simulink model "full_maneuver_platoon"  (R2022a)
settings: Solver=ode23t  StartTime=0.0  StopTime=300  FixedStep=0.1  MaxStep=0.01  RelTol=1e-3
InitFcn:
  | totalVehicles = 7;
  | if exist('vehStatesBus', 'var')==0
  | load vehBuses
  | end
  | if exist('vehErrorsBus', 'var')==0
  | load vehBuses
  | end
libraries: simulink x80, powerlib_meascontrol x16, autolibshared x7, dspsigops x4
(part 1 of 9)
settings Model: Creator=fvall  LastModifiedBy=fvall
settings SolverCC: AlgebraicLoopSolver=TrustRegion
settings DebuggingCC: ReadBeforeWriteMsg=DisableAll  WriteAfterWriteMsg=DisableAll  WriteAfterReadMsg=DisableAll  MultiTaskDSMMsg=none  UnconnectedInputMsg=warning  UnconnectedOutputMsg=warning  UnconnectedLineMsg=warning  SFMachineParentedDataDiag=warning
settings ModelReferenceCC: UpdateModelReferenceTargets=IfOutOfDate
settings SFSimCC: SFSimEcho=off  CustomCodeUndefinedFunction=UseInterfaceOnly

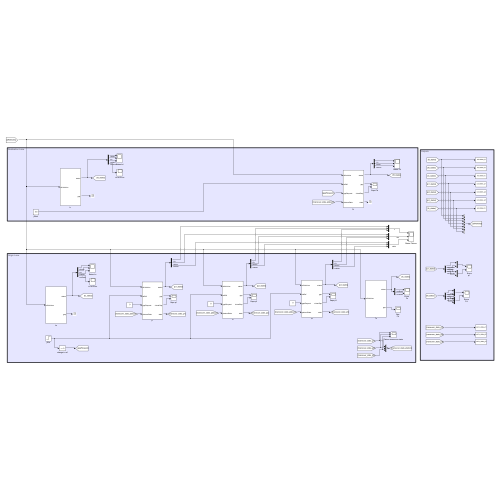
[thumbnail: Simulink's stored preview of the top-level diagram]
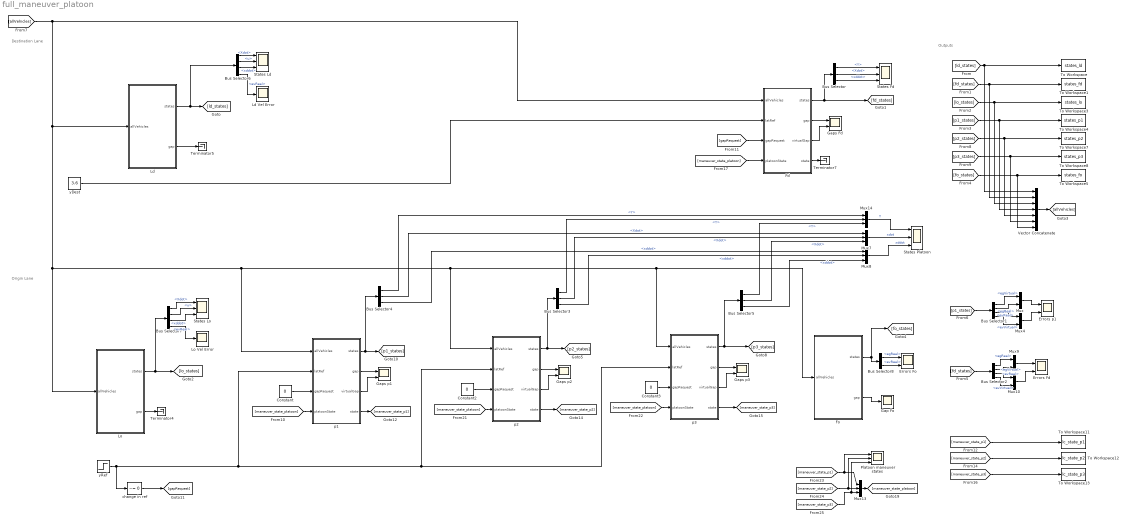
== system full_maneuver_platoon ==
  note: Destination Lane
  note: Outputs
  note: Origin Lane
  Bus Selector{,3..5} (4 alike) : BusSelector  OutputSignals=Y,Xdot,xddot
  Bus Selector1 : BusSelector  OutputSignals=egVirtual,egReal,evReal,evVirtual
  Bus Selector2 : BusSelector  OutputSignals=egReal,egVirtual,evReal,evVirtual
  Bus Selector6 : BusSelector  OutputSignals=Xdot,u,xddot,evReal
  Bus Selector7 : BusSelector  OutputSignals=Xdot,u,xddot,evReal
  Bus Selector8 : BusSelector  OutputSignals=egReal,evReal
  Constant : Constant  Value=0
  Constant2 : Constant  Value=0
  Constant3 : Constant  Value=0
  Errors Fd : Scope  NumInputPorts=2
  Errors Fo : Scope  NumInputPorts=2
  Errors p1 : Scope  NumInputPorts=2
  Fd : Subsystem  mask{m=2000, lf=2.5, lr=2.5, maxAcceleration=3, minAcceleration=-8, maxJerk=50, minJerk=-50, maxDelta=0.43633, maxDeltaDot=0.16406, freeFlowVel=30, posInPlatoon=1, tau=0.5, A=[0 1 20 0;0 -2.3 0 -21.4;0 0 0 1;0 -0.7 0 -7.6], B=[0;24;0;36], C=[1 0 0 0;0 1 0 0;0 0 1 0;0 0 0 1], x0=129.8137, vx0=25, y0=3.6, h=2.1778, d0=0.01134, minGapError=-100, maxGapError=Inf, velFilterGain=10, Kd=0.45918, Kp=0.045918, Ki=0, Ka=0.25255, Kdd=0.025255, velKi=0.11304, velKp=0.54492, velKd=0.07454, hFilterGain=0.3, hFilterSaturation=Inf, vMin=16.25, maxComfAccel=0.5, minComfAccel=-0.5, maxComfJerk=10, minComfJerk=-10, strategyChoice=leaderFirstInvert, hLC=2.2978, d0LC=0.01134, Klat=[0.0363636363636331 0.000980533179898461 1.32121212121203 0.0854574223245029], L=[3 1 20 0;0 3.7 0 -21.4;0 0 12 1;0 -0.7 0 10.4]}
      mask prompts: m "autoblks_shared:autoblkVehBody3DofLat:blkPrm_m"; lf "autoblks_shared:autoblkVehBody3DofLat:blkPrm_a"; lr "autoblks_shared:autoblkVehBody3DofLat:blkPrm_b"; maxAcceleration "Max Acceleration"; minAcceleration "Min Acceleration"; maxJerk "Max Jerk"; minJerk "Min Jerk"; maxDelta "Max Delta"; maxDeltaDot "Max Delta Dot"; freeFlowVel "Free Flow Velocity"; posInPlatoon "Position in Platoon"; tau "Actuator Lag"; x0 "autoblks_shared:autoblkVehBody3DofLat:blkPrm_X_o"; vx0 "autoblks_shared:autoblkVehBody3DofLat:blkPrm_xdot_o"; y0 "autoblks_shared:autoblkVehBody3DofLat:blkPrm_Y_o"; h "Time Headway"; d0 "Standstill Gap"; minGapError "Min Gap Error"; maxGapError "Max Gap Error"; velFilterGain "Velocity Filter Gain"; hFilterGain "Headway Filter Gain"; hFilterSaturation "Headway Filter Saturation"; vMin "Min Velocity"; maxComfAccel "Max Comf Accel"; minComfAccel "Min Comf Accel"; maxComfJerk "Max Comf Jerk"; minComfJerk "Min Comf Jerk"; strategyChoice "Lane Change Strategy"; hLC "Time Headway LC"; d0LC "Standstill Gap LC"; Klat "Lat Controller Gain"; L "Observer Gain"
      mask TypeOptions m: Vehicle Body 3DOF Single Track/m
      mask TypeOptions lf: Vehicle Body 3DOF Single Track/a
      mask TypeOptions lr: Vehicle Body 3DOF Single Track/b
      mask TypeOptions maxDelta: Lateral Control/Saturation/UpperLimit
      mask TypeOptions maxDeltaDot: Lateral Control/Rate Limiter/RisingSlewLimit
      mask TypeOptions posInPlatoon: posInPlatoon/Value
      mask TypeOptions A:
      | Lateral Control/Full State
      | Observer/Gain3/Gain
      mask TypeOptions B:
      | Lateral Control/Full State
      | Observer/Gain/Gain
      mask TypeOptions C:
      | Lateral Control/Full State
      | Observer/Gain1/Gain
      mask TypeOptions x0: Vehicle Body 3DOF Single Track/X_o
      mask TypeOptions vx0: Vehicle Body 3DOF Single Track/xdot_o
      mask TypeOptions y0: Vehicle Body 3DOF Single Track/Y_o
      mask TypeOptions strategyChoice: Lane Change Strategy/LabelModeActiveChoice
      mask TypeOptions Klat: Lateral Control/Gain1/Gain
      mask TypeOptions L:
      | Lateral Control/Full State
      | Observer/Gain2/Gain
      mask DialogControl DescGroupVar Prompt: 3DOF Vehicle with ACC
      mask DialogControl DescTextVar Prompt: Vehicle with ACC. The vehicle model is Simulink's 3DOF single track vehicle body. The controller is a PID with constant headway including headway error saturation and filtered leader velocity.
      mask DialogControl VehParams Prompt: Vehicle Parameters
      mask DialogControl m Prompt: Vehicle mass, m [kg]:
      mask DialogControl lf Prompt: Longitudinal distance from center of mass to front axle, a [m]:
      mask DialogControl lr Prompt: Longitudinal distance from center of mass to rear axle, b [m]:
      mask DialogControl latLinearModel Prompt: Lat Linear Model
      mask DialogControl InitStates Prompt: Initial State
      mask DialogControl x0 Prompt: Initial inertial frame longitudinal position, X_o [m]:
      mask DialogControl vx0 Prompt: Initial longitudinal velocity, xdot_o [m/s]:
      mask DialogControl y0 Prompt: Initial inertial frame lateral displacement, Y_o [m]:
      mask DialogControl Container3 Prompt: Veh Following Parameters
      mask DialogControl ComfortConstraints Prompt: Comfort Constraints
      mask DialogControl LCParams Prompt: Lane Change Params
  Fo : Subsystem  mask{m=2000, lf=2.5, lr=2.5, maxAcceleration=3, minAcceleration=-8, maxJerk=50, minJerk=-50, freeFlowVel=30, tau=0.5, x0=0, vx0=20, y0=0, h=2.1778, d0=0.01134, minGapError=-100, maxGapError=Inf, velFilterGain=10, Kd=0.45918, Kp=0.045918, Ki=0, Ka=0.25255, Kdd=0.025255, velKi=0.11304, velKp=0.54492, velKd=0.07454, hFilterGain=0.3, hFilterSaturation=Inf, vMin=13, maxComfAccel=0.5, minComfAccel=-0.5, maxComfJerk=10, minComfJerk=-10, hLC=2.2978, d0LC=0.01134}
      mask prompts: m "autoblks_shared:autoblkVehBody3DofLat:blkPrm_m"; lf "autoblks_shared:autoblkVehBody3DofLat:blkPrm_a"; lr "autoblks_shared:autoblkVehBody3DofLat:blkPrm_b"; maxAcceleration "Max Acceleration"; minAcceleration "Min Acceleration"; maxJerk "Max Jerk"; minJerk "Min Jerk"; freeFlowVel "Free Flow Velocity"; tau "Actuator Lag"; x0 "autoblks_shared:autoblkVehBody3DofLat:blkPrm_X_o"; vx0 "autoblks_shared:autoblkVehBody3DofLat:blkPrm_xdot_o"; y0 "autoblks_shared:autoblkVehBody3DofLat:blkPrm_Y_o"; h "Time Headway"; d0 "Standstill Gap"; minGapError "Min Gap Error"; maxGapError "Max Gap Error"; velFilterGain "Velocity Filter Gain"; hFilterGain "Headway Filter Gain"; hFilterSaturation "Headway Filter Saturation"; vMin "Min Velocity"; maxComfAccel "Max Comf Accel"; minComfAccel "Min Comf Accel"; maxComfJerk "Max Comf Jerk"; minComfJerk "Min Comf Jerk"; hLC "Time Headway LC"; d0LC "Standstill Gap LC"
      mask TypeOptions m: Vehicle Body 3DOF Single Track/m
      mask TypeOptions lf: Vehicle Body 3DOF Single Track/a
      mask TypeOptions lr: Vehicle Body 3DOF Single Track/b
      mask TypeOptions x0: Vehicle Body 3DOF Single Track/X_o
      mask TypeOptions vx0: Vehicle Body 3DOF Single Track/xdot_o
      mask TypeOptions y0: Vehicle Body 3DOF Single Track/Y_o
      mask DialogControl DescGroupVar Prompt: 3DOF Vehicle with ACC
      mask DialogControl DescTextVar Prompt: Vehicle with ACC. The vehicle model is Simulink's 3DOF single track vehicle body. The controller is a PID with constant headway including headway error saturation and filtered leader velocity.
      mask DialogControl VehParams Prompt: Vehicle Parameters
      mask DialogControl m Prompt: Vehicle mass, m [kg]:
      mask DialogControl lf Prompt: Longitudinal distance from center of mass to front axle, a [m]:
      mask DialogControl lr Prompt: Longitudinal distance from center of mass to rear axle, b [m]:
      mask DialogControl InitStates Prompt: Initial State
      mask DialogControl x0 Prompt: Initial inertial frame longitudinal position, X_o [m]:
      mask DialogControl vx0 Prompt: Initial longitudinal velocity, xdot_o [m/s]:
      mask DialogControl y0 Prompt: Initial inertial frame lateral displacement, Y_o [m]:
      mask DialogControl Container3 Prompt: Veh Following Parameters
      mask DialogControl ComfortConstraints Prompt: Comfort Constraints
      mask DialogControl LaneChangeParams Prompt: Lane Change Params
  Gap Fo : Scope
  Gaps Fd : Scope  NumInputPorts=2
  Gaps p1 : Scope  NumInputPorts=2
  Gaps p2 : Scope  NumInputPorts=2
  Gaps p3 : Scope  NumInputPorts=2
  Ld : Subsystem  mask{m=2000, lf=2.5, lr=2.5, maxAcceleration=3, minAcceleration=-8, maxJerk=50, minJerk=-50, freeFlowVel=25, tau=0.5, x0=189.2704, vx0=25, y0=3.6, h=0.30281, d0=0.01134, minGapError=-100, maxGapError=Inf, velFilterGain=10, Kd=3.3024, Kp=0.33024, Ki=0, Ka=1.8163, Kdd=0.18163, velKi=0.11304, velKp=0.54492, velKd=0.07454, hFilterGain=0.3, hFilterSaturation=Inf, vMin=16.25, maxComfAccel=0.5, minComfAccel=-0.5, maxComfJerk=10, minComfJerk=-10, hLC=1.8025, d0LC=0.01134}
      mask prompts: m "autoblks_shared:autoblkVehBody3DofLat:blkPrm_m"; lf "autoblks_shared:autoblkVehBody3DofLat:blkPrm_a"; lr "autoblks_shared:autoblkVehBody3DofLat:blkPrm_b"; maxAcceleration "Max Acceleration"; minAcceleration "Min Acceleration"; maxJerk "Max Jerk"; minJerk "Min Jerk"; freeFlowVel "Free Flow Velocity"; tau "Actuator Lag"; x0 "autoblks_shared:autoblkVehBody3DofLat:blkPrm_X_o"; vx0 "autoblks_shared:autoblkVehBody3DofLat:blkPrm_xdot_o"; y0 "autoblks_shared:autoblkVehBody3DofLat:blkPrm_Y_o"; h "Time Headway"; d0 "Standstill Gap"; minGapError "Min Gap Error"; maxGapError "Max Gap Error"; velFilterGain "Velocity Filter Gain"; hFilterGain "Headway Filter Gain"; hFilterSaturation "Headway Filter Saturation"; vMin "Min Velocity"; maxComfAccel "Max Comf Accel"; minComfAccel "Min Comf Accel"; maxComfJerk "Max Comf Jerk"; minComfJerk "Min Comf Jerk"; hLC "Time Headway LC"; d0LC "Standstill Gap LC"
      mask TypeOptions m: Vehicle Body 3DOF Single Track/m
      mask TypeOptions lf: Vehicle Body 3DOF Single Track/a
      mask TypeOptions lr: Vehicle Body 3DOF Single Track/b
      mask TypeOptions x0: Vehicle Body 3DOF Single Track/X_o
      mask TypeOptions vx0: Vehicle Body 3DOF Single Track/xdot_o
      mask TypeOptions y0: Vehicle Body 3DOF Single Track/Y_o
      mask DialogControl DescGroupVar Prompt: 3DOF Vehicle with ACC
      mask DialogControl DescTextVar Prompt: Vehicle with ACC. The vehicle model is Simulink's 3DOF single track vehicle body. The controller is a PID with constant headway including headway error saturation and filtered leader velocity.
      mask DialogControl VehParams Prompt: Vehicle Parameters
      mask DialogControl m Prompt: Vehicle mass, m [kg]:
      mask DialogControl lf Prompt: Longitudinal distance from center of mass to front axle, a [m]:
      mask DialogControl lr Prompt: Longitudinal distance from center of mass to rear axle, b [m]:
      mask DialogControl InitStates Prompt: Initial State
      mask DialogControl x0 Prompt: Initial inertial frame longitudinal position, X_o [m]:
      mask DialogControl vx0 Prompt: Initial longitudinal velocity, xdot_o [m/s]:
      mask DialogControl y0 Prompt: Initial inertial frame lateral displacement, Y_o [m]:
      mask DialogControl Container3 Prompt: Veh Following Parameters
      mask DialogControl ComfortConstraints Prompt: Comfort Constraints
      mask DialogControl LaneChangeParams Prompt: Lane Change Params
  Ld Vel Error : Scope
  Lo : Subsystem  mask{m=2000, lf=2.5, lr=2.5, maxAcceleration=3, minAcceleration=-8, maxJerk=50, minJerk=-50, freeFlowVel=20, tau=0.5, x0=194.2704, vx0=20, y0=0, h=0.30281, d0=0.01134, minGapError=-100, maxGapError=Inf, velFilterGain=10, Kd=3.3024, Kp=0.33024, Ki=0, Ka=1.8163, Kdd=0.18163, velKi=0.11304, velKp=0.54492, velKd=0.07454, hFilterGain=0.3, hFilterSaturation=Inf, vMin=13, maxComfAccel=0.5, minComfAccel=-0.5, maxComfJerk=10, minComfJerk=-10, hLC=1.49, d0LC=0.01134}
      mask prompts: m "autoblks_shared:autoblkVehBody3DofLat:blkPrm_m"; lf "autoblks_shared:autoblkVehBody3DofLat:blkPrm_a"; lr "autoblks_shared:autoblkVehBody3DofLat:blkPrm_b"; maxAcceleration "Max Acceleration"; minAcceleration "Min Acceleration"; maxJerk "Max Jerk"; minJerk "Min Jerk"; freeFlowVel "Free Flow Velocity"; tau "Actuator Lag"; x0 "autoblks_shared:autoblkVehBody3DofLat:blkPrm_X_o"; vx0 "autoblks_shared:autoblkVehBody3DofLat:blkPrm_xdot_o"; y0 "autoblks_shared:autoblkVehBody3DofLat:blkPrm_Y_o"; h "Time Headway"; d0 "Standstill Gap"; minGapError "Min Gap Error"; maxGapError "Max Gap Error"; velFilterGain "Velocity Filter Gain"; hFilterGain "Headway Filter Gain"; hFilterSaturation "Headway Filter Saturation"; vMin "Min Velocity"; maxComfAccel "Max Comf Accel"; minComfAccel "Min Comf Accel"; maxComfJerk "Max Comf Jerk"; minComfJerk "Min Comf Jerk"; hLC "Time Headway LC"; d0LC "Standstill Gap LC"
      mask TypeOptions m: Vehicle Body 3DOF Single Track/m
      mask TypeOptions lf: Vehicle Body 3DOF Single Track/a
      mask TypeOptions lr: Vehicle Body 3DOF Single Track/b
      mask TypeOptions x0: Vehicle Body 3DOF Single Track/X_o
      mask TypeOptions vx0: Vehicle Body 3DOF Single Track/xdot_o
      mask TypeOptions y0: Vehicle Body 3DOF Single Track/Y_o
      mask DialogControl DescGroupVar Prompt: 3DOF Vehicle with ACC
      mask DialogControl DescTextVar Prompt: Vehicle with ACC. The vehicle model is Simulink's 3DOF single track vehicle body. The controller is a PID with constant headway including headway error saturation and filtered leader velocity.
      mask DialogControl VehParams Prompt: Vehicle Parameters
      mask DialogControl m Prompt: Vehicle mass, m [kg]:
      mask DialogControl lf Prompt: Longitudinal distance from center of mass to front axle, a [m]:
      mask DialogControl lr Prompt: Longitudinal distance from center of mass to rear axle, b [m]:
      mask DialogControl InitStates Prompt: Initial State
      mask DialogControl x0 Prompt: Initial inertial frame longitudinal position, X_o [m]:
      mask DialogControl vx0 Prompt: Initial longitudinal velocity, xdot_o [m/s]:
      mask DialogControl y0 Prompt: Initial inertial frame lateral displacement, Y_o [m]:
      mask DialogControl Container3 Prompt: Veh Following Parameters
      mask DialogControl ComfortConstraints Prompt: Comfort Constraints
      mask DialogControl LaneChangeParams Prompt: Lane Change Params
  Lo Vel Error : Scope
  Mux{,4,9..10} (4 alike) : Mux  Inputs=2
  Mux{7..8,13..14} (4 alike) : Mux  Inputs=3
  Platoon maneuver states : Scope  NumInputPorts=3
  States Fd : Scope  NumInputPorts=3
  States Ld : Scope  NumInputPorts=3
  States Lo : Scope  NumInputPorts=3
  States Platoon : Scope  NumInputPorts=3
  Terminator4 : Terminator
  Terminator5 : Terminator
  Terminator7 : Terminator
  To Workspace : ToWorkspace  VariableName=states_ld  SaveFormat=Timeseries  SampleTime=-1
  To Workspace1 : ToWorkspace  VariableName=states_fd  SaveFormat=Timeseries  SampleTime=-1
  To Workspace11 : ToWorkspace  VariableName=lc_state_p1  SaveFormat=Timeseries  SampleTime=-1
  To Workspace12 : ToWorkspace  VariableName=lc_state_p2  SaveFormat=Timeseries  SampleTime=-1
  To Workspace13 : ToWorkspace  VariableName=lc_state_p3  SaveFormat=Timeseries  SampleTime=-1
  To Workspace3 : ToWorkspace  VariableName=states_lo  SaveFormat=Timeseries  SampleTime=-1
  To Workspace4 : ToWorkspace  VariableName=states_p1  SaveFormat=Timeseries  SampleTime=-1
  To Workspace5 : ToWorkspace  VariableName=states_fo  SaveFormat=Timeseries  SampleTime=-1
  To Workspace7 : ToWorkspace  VariableName=states_p2  SaveFormat=Timeseries  SampleTime=-1
  To Workspace8 : ToWorkspace  VariableName=states_p3  SaveFormat=Timeseries  SampleTime=-1
  Vector Concatenate : Concatenate  NumInputs=7
  change in ref : simulink/Logic and Bit Operations/Compare To Constant  relop=~=  const=0  OutDataTypeStr=boolean
  p1 : Subsystem  mask{m=2000, lf=2.5, lr=2.5, maxAcceleration=3, minAcceleration=-8, maxJerk=50, minJerk=-50, maxDelta=0.43633, maxDeltaDot=0.16406, freeFlowVel=30, posInPlatoon=1, tau=0.5, A=[0 1 20 0;0 -2.3 0 -21.4;0 0 0 1;0 -0.7 0 -7.6], B=[0;24;0;36], C=[1 0 0 0;0 1 0 0;0 0 1 0;0 0 0 1], x0=145.7028, vx0=20, y0=0, h=2.1778, d0=0.01134, minGapError=-100, maxGapError=Inf, velFilterGain=10, Kd=0.45918, Kp=0.045918, Ki=0, Ka=0.25255, Kdd=0.025255, velKi=0.11304, velKp=0.54492, velKd=0.07454, hFilterGain=0.3, hFilterSaturation=Inf, vMin=13, maxComfAccel=0.5, minComfAccel=-0.5, maxComfJerk=10, minComfJerk=-10, strategyChoice=leaderFirstInvert, hLC=2.2978, d0LC=0.01134, Klat=[0.0363636363636331 0.000980533179898461 1.32121212121203 0.0854574223245029], L=[3 1 20 0;0 3.7 0 -21.4;0 0 12 1;0 -0.7 0 10.4]}
      mask prompts: m "autoblks_shared:autoblkVehBody3DofLat:blkPrm_m"; lf "autoblks_shared:autoblkVehBody3DofLat:blkPrm_a"; lr "autoblks_shared:autoblkVehBody3DofLat:blkPrm_b"; maxAcceleration "Max Acceleration"; minAcceleration "Min Acceleration"; maxJerk "Max Jerk"; minJerk "Min Jerk"; maxDelta "Max Delta"; maxDeltaDot "Max Delta Dot"; freeFlowVel "Free Flow Velocity"; posInPlatoon "Position in Platoon"; tau "Actuator Lag"; x0 "autoblks_shared:autoblkVehBody3DofLat:blkPrm_X_o"; vx0 "autoblks_shared:autoblkVehBody3DofLat:blkPrm_xdot_o"; y0 "autoblks_shared:autoblkVehBody3DofLat:blkPrm_Y_o"; h "Time Headway"; d0 "Standstill Gap"; minGapError "Min Gap Error"; maxGapError "Max Gap Error"; velFilterGain "Velocity Filter Gain"; hFilterGain "Headway Filter Gain"; hFilterSaturation "Headway Filter Saturation"; vMin "Min Velocity"; maxComfAccel "Max Comf Accel"; minComfAccel "Min Comf Accel"; maxComfJerk "Max Comf Jerk"; minComfJerk "Min Comf Jerk"; strategyChoice "Lane Change Strategy"; hLC "Time Headway LC"; d0LC "Standstill Gap LC"; Klat "Lat Controller Gain"; L "Observer Gain"
      mask TypeOptions m: Vehicle Body 3DOF Single Track/m
      mask TypeOptions lf: Vehicle Body 3DOF Single Track/a
      mask TypeOptions lr: Vehicle Body 3DOF Single Track/b
      mask TypeOptions maxDelta: Lateral Control/Saturation/UpperLimit
      mask TypeOptions maxDeltaDot: Lateral Control/Rate Limiter/RisingSlewLimit
      mask TypeOptions posInPlatoon: posInPlatoon/Value
      mask TypeOptions A:
      | Lateral Control/Full State
      | Observer/Gain3/Gain
      mask TypeOptions B:
      | Lateral Control/Full State
      | Observer/Gain/Gain
      mask TypeOptions C:
      | Lateral Control/Full State
      | Observer/Gain1/Gain
      mask TypeOptions x0: Vehicle Body 3DOF Single Track/X_o
      mask TypeOptions vx0: Vehicle Body 3DOF Single Track/xdot_o
      mask TypeOptions y0: Vehicle Body 3DOF Single Track/Y_o
      mask TypeOptions strategyChoice: Lane Change Strategy/LabelModeActiveChoice
      mask TypeOptions Klat: Lateral Control/Gain1/Gain
      mask TypeOptions L:
      | Lateral Control/Full State
      | Observer/Gain2/Gain
      mask DialogControl DescGroupVar Prompt: 3DOF Vehicle with ACC
      mask DialogControl DescTextVar Prompt: Vehicle with ACC. The vehicle model is Simulink's 3DOF single track vehicle body. The controller is a PID with constant headway including headway error saturation and filtered leader velocity.
      mask DialogControl VehParams Prompt: Vehicle Parameters
      mask DialogControl m Prompt: Vehicle mass, m [kg]:
      mask DialogControl lf Prompt: Longitudinal distance from center of mass to front axle, a [m]:
      mask DialogControl lr Prompt: Longitudinal distance from center of mass to rear axle, b [m]:
      mask DialogControl latLinearModel Prompt: Lat Linear Model
      mask DialogControl InitStates Prompt: Initial State
      mask DialogControl x0 Prompt: Initial inertial frame longitudinal position, X_o [m]:
      mask DialogControl vx0 Prompt: Initial longitudinal velocity, xdot_o [m/s]:
      mask DialogControl y0 Prompt: Initial inertial frame lateral displacement, Y_o [m]:
      mask DialogControl Container3 Prompt: Veh Following Parameters
      mask DialogControl ComfortConstraints Prompt: Comfort Constraints
      mask DialogControl LCParams Prompt: Lane Change Params
  p2 : Subsystem  mask{m=2000, lf=2.5, lr=2.5, maxAcceleration=3, minAcceleration=-8, maxJerk=50, minJerk=-50, maxDelta=0.43633, maxDeltaDot=0.16406, freeFlowVel=30, posInPlatoon=2, tau=0.5, A=[0 1 20 0;0 -2.3 0 -21.4;0 0 0 1;0 -0.7 0 -7.6], B=[0;24;0;36], C=[1 0 0 0;0 1 0 0;0 0 1 0;0 0 0 1], x0=97.1352, vx0=20, y0=0, h=2.1778, d0=0.01134, minGapError=-100, maxGapError=Inf, velFilterGain=10, Kd=0.45918, Kp=0.045918, Ki=0, Ka=0.25255, Kdd=0.025255, velKi=0.11304, velKp=0.54492, velKd=0.07454, hFilterGain=0.3, hFilterSaturation=Inf, vMin=13, maxComfAccel=0.5, minComfAccel=-0.5, maxComfJerk=10, minComfJerk=-10, strategyChoice=leaderFirstInvert, hLC=2.2978, d0LC=0.01134, Klat=[0.0363636363636331 0.000980533179898461 1.32121212121203 0.0854574223245029], L=[3 1 20 0;0 3.7 0 -21.4;0 0 12 1;0 -0.7 0 10.4]}
      mask prompts: m "autoblks_shared:autoblkVehBody3DofLat:blkPrm_m"; lf "autoblks_shared:autoblkVehBody3DofLat:blkPrm_a"; lr "autoblks_shared:autoblkVehBody3DofLat:blkPrm_b"; maxAcceleration "Max Acceleration"; minAcceleration "Min Acceleration"; maxJerk "Max Jerk"; minJerk "Min Jerk"; maxDelta "Max Delta"; maxDeltaDot "Max Delta Dot"; freeFlowVel "Free Flow Velocity"; posInPlatoon "Position in Platoon"; tau "Actuator Lag"; x0 "autoblks_shared:autoblkVehBody3DofLat:blkPrm_X_o"; vx0 "autoblks_shared:autoblkVehBody3DofLat:blkPrm_xdot_o"; y0 "autoblks_shared:autoblkVehBody3DofLat:blkPrm_Y_o"; h "Time Headway"; d0 "Standstill Gap"; minGapError "Min Gap Error"; maxGapError "Max Gap Error"; velFilterGain "Velocity Filter Gain"; hFilterGain "Headway Filter Gain"; hFilterSaturation "Headway Filter Saturation"; vMin "Min Velocity"; maxComfAccel "Max Comf Accel"; minComfAccel "Min Comf Accel"; maxComfJerk "Max Comf Jerk"; minComfJerk "Min Comf Jerk"; strategyChoice "Lane Change Strategy"; hLC "Time Headway LC"; d0LC "Standstill Gap LC"; Klat "Lat Controller Gain"; L "Observer Gain"
      mask TypeOptions m: Vehicle Body 3DOF Single Track/m
      mask TypeOptions lf: Vehicle Body 3DOF Single Track/a
      mask TypeOptions lr: Vehicle Body 3DOF Single Track/b
      mask TypeOptions maxDelta: Lateral Control/Saturation/UpperLimit
      mask TypeOptions maxDeltaDot: Lateral Control/Rate Limiter/RisingSlewLimit
      mask TypeOptions posInPlatoon: posInPlatoon/Value
      mask TypeOptions A:
      | Lateral Control/Full State
      | Observer/Gain3/Gain
      mask TypeOptions B:
      | Lateral Control/Full State
      | Observer/Gain/Gain
      mask TypeOptions C:
      | Lateral Control/Full State
      | Observer/Gain1/Gain
      mask TypeOptions x0: Vehicle Body 3DOF Single Track/X_o
      mask TypeOptions vx0: Vehicle Body 3DOF Single Track/xdot_o
      mask TypeOptions y0: Vehicle Body 3DOF Single Track/Y_o
      mask TypeOptions strategyChoice: Lane Change Strategy/LabelModeActiveChoice
      mask TypeOptions Klat: Lateral Control/Gain1/Gain
      mask TypeOptions L:
      | Lateral Control/Full State
      | Observer/Gain2/Gain
      mask DialogControl DescGroupVar Prompt: 3DOF Vehicle with ACC
      mask DialogControl DescTextVar Prompt: Vehicle with ACC. The vehicle model is Simulink's 3DOF single track vehicle body. The controller is a PID with constant headway including headway error saturation and filtered leader velocity.
      mask DialogControl VehParams Prompt: Vehicle Parameters
      mask DialogControl m Prompt: Vehicle mass, m [kg]:
      mask DialogControl lf Prompt: Longitudinal distance from center of mass to front axle, a [m]:
      mask DialogControl lr Prompt: Longitudinal distance from center of mass to rear axle, b [m]:
      mask DialogControl latLinearModel Prompt: Lat Linear Model
      mask DialogControl InitStates Prompt: Initial State
      mask DialogControl x0 Prompt: Initial inertial frame longitudinal position, X_o [m]:
      mask DialogControl vx0 Prompt: Initial longitudinal velocity, xdot_o [m/s]:
      mask DialogControl y0 Prompt: Initial inertial frame lateral displacement, Y_o [m]:
      mask DialogControl Container3 Prompt: Veh Following Parameters
      mask DialogControl ComfortConstraints Prompt: Comfort Constraints
      mask DialogControl LCParams Prompt: Lane Change Params
  p3 : Subsystem  mask{m=2000, lf=2.5, lr=2.5, maxAcceleration=3, minAcceleration=-8, maxJerk=50, minJerk=-50, maxDelta=0.43633, maxDeltaDot=0.16406, freeFlowVel=30, posInPlatoon=3, tau=0.5, A=[0 1 20 0;0 -2.3 0 -21.4;0 0 0 1;0 -0.7 0 -7.6], B=[0;24;0;36], C=[1 0 0 0;0 1 0 0;0 0 1 0;0 0 0 1], x0=48.5676, vx0=20, y0=0, h=2.1778, d0=0.01134, minGapError=-100, maxGapError=Inf, velFilterGain=10, Kd=0.45918, Kp=0.045918, Ki=0, Ka=0.25255, Kdd=0.025255, velKi=0.11304, velKp=0.54492, velKd=0.07454, hFilterGain=0.3, hFilterSaturation=Inf, vMin=13, maxComfAccel=0.5, minComfAccel=-0.5, maxComfJerk=10, minComfJerk=-10, strategyChoice=leaderFirstInvert, hLC=2.2978, d0LC=0.01134, Klat=[0.0363636363636331 0.000980533179898461 1.32121212121203 0.0854574223245029], L=[3 1 20 0;0 3.7 0 -21.4;0 0 12 1;0 -0.7 0 10.4]}
      mask prompts: m "autoblks_shared:autoblkVehBody3DofLat:blkPrm_m"; lf "autoblks_shared:autoblkVehBody3DofLat:blkPrm_a"; lr "autoblks_shared:autoblkVehBody3DofLat:blkPrm_b"; maxAcceleration "Max Acceleration"; minAcceleration "Min Acceleration"; maxJerk "Max Jerk"; minJerk "Min Jerk"; maxDelta "Max Delta"; maxDeltaDot "Max Delta Dot"; freeFlowVel "Free Flow Velocity"; posInPlatoon "Position in Platoon"; tau "Actuator Lag"; x0 "autoblks_shared:autoblkVehBody3DofLat:blkPrm_X_o"; vx0 "autoblks_shared:autoblkVehBody3DofLat:blkPrm_xdot_o"; y0 "autoblks_shared:autoblkVehBody3DofLat:blkPrm_Y_o"; h "Time Headway"; d0 "Standstill Gap"; minGapError "Min Gap Error"; maxGapError "Max Gap Error"; velFilterGain "Velocity Filter Gain"; hFilterGain "Headway Filter Gain"; hFilterSaturation "Headway Filter Saturation"; vMin "Min Velocity"; maxComfAccel "Max Comf Accel"; minComfAccel "Min Comf Accel"; maxComfJerk "Max Comf Jerk"; minComfJerk "Min Comf Jerk"; strategyChoice "Lane Change Strategy"; hLC "Time Headway LC"; d0LC "Standstill Gap LC"; Klat "Lat Controller Gain"; L "Observer Gain"
      mask TypeOptions m: Vehicle Body 3DOF Single Track/m
      mask TypeOptions lf: Vehicle Body 3DOF Single Track/a
      mask TypeOptions lr: Vehicle Body 3DOF Single Track/b
      mask TypeOptions maxDelta: Lateral Control/Saturation/UpperLimit
      mask TypeOptions maxDeltaDot: Lateral Control/Rate Limiter/RisingSlewLimit
      mask TypeOptions posInPlatoon: posInPlatoon/Value
      mask TypeOptions A:
      | Lateral Control/Full State
      | Observer/Gain3/Gain
      mask TypeOptions B:
      | Lateral Control/Full State
      | Observer/Gain/Gain
      mask TypeOptions C:
      | Lateral Control/Full State
      | Observer/Gain1/Gain
      mask TypeOptions x0: Vehicle Body 3DOF Single Track/X_o
      mask TypeOptions vx0: Vehicle Body 3DOF Single Track/xdot_o
      mask TypeOptions y0: Vehicle Body 3DOF Single Track/Y_o
      mask TypeOptions strategyChoice: Lane Change Strategy/LabelModeActiveChoice
      mask TypeOptions Klat: Lateral Control/Gain1/Gain
      mask TypeOptions L:
      | Lateral Control/Full State
      | Observer/Gain2/Gain
      mask DialogControl DescGroupVar Prompt: 3DOF Vehicle with ACC
      mask DialogControl DescTextVar Prompt: Vehicle with ACC. The vehicle model is Simulink's 3DOF single track vehicle body. The controller is a PID with constant headway including headway error saturation and filtered leader velocity.
      mask DialogControl VehParams Prompt: Vehicle Parameters
      mask DialogControl m Prompt: Vehicle mass, m [kg]:
      mask DialogControl lf Prompt: Longitudinal distance from center of mass to front axle, a [m]:
      mask DialogControl lr Prompt: Longitudinal distance from center of mass to rear axle, b [m]:
      mask DialogControl latLinearModel Prompt: Lat Linear Model
      mask DialogControl InitStates Prompt: Initial State
      mask DialogControl x0 Prompt: Initial inertial frame longitudinal position, X_o [m]:
      mask DialogControl vx0 Prompt: Initial longitudinal velocity, xdot_o [m/s]:
      mask DialogControl y0 Prompt: Initial inertial frame lateral displacement, Y_o [m]:
      mask DialogControl Container3 Prompt: Veh Following Parameters
      mask DialogControl ComfortConstraints Prompt: Comfort Constraints
      mask DialogControl LCParams Prompt: Lane Change Params
  yDest : Constant  Value=3.6
  yRef : Step  Time=2  After=3.6  SampleTime=0
  wires:
  [p1_states] -> Bus Selector1/1
  p1/3(virtualGap) -> Gaps p1/2
  [fo_states] -> To Workspace5/1, Vector Concatenate/7
  [ld_states] -> To Workspace/1, Vector Concatenate/1
  [p1_states] -> Vector Concatenate/4, To Workspace4/1
  [fd_states] -> Bus Selector2/1
  change in ref/1 -> [gapRequest]
  Mux9/1 -> Errors Fd/1
  Mux10/1 -> Errors Fd/2
  p1/1(states) -> Bus Selector4/1, [p1_states]
  [lo_states] -> To Workspace3/1, Vector Concatenate/3
  Bus Selector/2 -> States Fd/2  "<Xdot>"
  p1/2(gap) -> Gaps p1/1
  [fd_states] -> To Workspace1/1, Vector Concatenate/2
  Bus Selector/3 -> States Fd/3  "<xddot>"
  Fd/3(virtualGap) -> Gaps Fd/2
  Fd/2(gap) -> Gaps Fd/1
  Fd/1(states) -> [fd_states], Bus Selector/1
  Fd/4(state) -> Terminator7/1
  Bus Selector4/2 -> Mux7/1  "<Xdot>"
  yRef/1 -> change in ref/1, p1/2(latRef), p3/2(latRef), p2/2(latRef)
  yDest/1 -> Fd/2(latRef)
  Bus Selector/1 -> States Fd/1  "<Y>"
  [allVehicles] -> Fd/1(allVehicles), Ld/1(allVehicles), Lo/1(allVehicles), p1/1(allVehicles), p2/1(allVehicles), p3/1(allVehicles), Fo/1(allVehicles)
  Vector Concatenate/1 -> [allVehicles]
  p2/2(gap) -> Gaps p2/1
  p2/3(virtualGap) -> Gaps p2/2
  p2/1(states) -> Bus Selector3/1, [p2_states]
  Bus Selector3/2 -> Mux7/2  "<Xdot>"
  Bus Selector3/1 -> Mux14/2  "<Y>"
  Bus Selector5/2 -> Mux7/3  "<Xdot>"
  Bus Selector5/1 -> Mux14/3  "<Y>"
  p3/1(states) -> Bus Selector5/1, [p3_states]
  p3/3(virtualGap) -> Gaps p3/2
  p3/2(gap) -> Gaps p3/1
  [p2_states] -> Vector Concatenate/5, To Workspace7/1
  [p3_states] -> Vector Concatenate/6, To Workspace8/1
  Mux7/1 -> States Platoon/2  "xdot"
  Mux8/1 -> States Platoon/3  "xddot"
  [gapRequest] -> Fd/3(gapRequest)
  p1/4(state) -> [maneuver_state_p1]
  p2/4(state) -> [maneuver_state_p2]
  p3/4(state) -> [maneuver_state_p3]
  Constant/1 -> p1/3(gapRequest)
  Constant2/1 -> p2/3(gapRequest)
  Constant3/1 -> p3/3(gapRequest)
  [maneuver_state_platoon] -> p1/4(platoonState)
  [maneuver_state_platoon] -> p2/4(platoonState)
  [maneuver_state_platoon] -> p3/4(platoonState)
  [maneuver_state_platoon] -> Fd/4(platoonState)
  [maneuver_state_p2] -> Platoon maneuver states/2, Mux13/2
  [maneuver_state_p1] -> Mux13/1, Platoon maneuver states/1
  [maneuver_state_p3] -> Platoon maneuver states/3, Mux13/3
  Mux13/1 -> [maneuver_state_platoon]
  Bus Selector4/1 -> Mux14/1  "<Y>"
  Mux14/1 -> States Platoon/1  "Y"
  [maneuver_state_p1] -> To Workspace11/1
  [maneuver_state_p3] -> To Workspace13/1
  [maneuver_state_p2] -> To Workspace12/1
  Bus Selector1/2 -> Mux/2  "<egReal>"
  Bus Selector1/1 -> Mux/1  "<egVirtual>"
  Mux/1 -> Errors p1/1
  Bus Selector1/3 -> Mux4/1  "<evReal>"
  Bus Selector1/4 -> Mux4/2  "<evVirtual>"
  Mux4/1 -> Errors p1/2
  Bus Selector2/1 -> Mux9/1  "<egReal>"
  Bus Selector2/2 -> Mux9/2  "<egVirtual>"
  Bus Selector2/3 -> Mux10/1  "<evReal>"
  Bus Selector2/4 -> Mux10/2  "<evVirtual>"
  Bus Selector6/1 -> States Ld/1  "<Xdot>"
  Bus Selector6/2 -> States Ld/2  "<u>"
  Ld/1(states) -> Bus Selector6/1, [ld_states]
  Bus Selector6/3 -> States Ld/3  "<xddot>"
  Ld/2(gap) -> Terminator5/1
  Lo/1(states) -> Bus Selector7/1, [lo_states]
  Bus Selector7/3 -> States Lo/3  "<xddot>"
  Bus Selector7/2 -> States Lo/2  "<u>"
  Bus Selector7/1 -> States Lo/1  "<Xdot>"
  Lo/2(gap) -> Terminator4/1
  Fo/2(gap) -> Gap Fo/1
  Bus Selector8/1 -> Errors Fo/1  "<egReal>"
  Fo/1(states) -> Bus Selector8/1, [fo_states]
  Bus Selector4/3 -> Mux8/1  "<xddot>"
  Bus Selector3/3 -> Mux8/2  "<xddot>"
  Bus Selector5/3 -> Mux8/3  "<xddot>"
  Bus Selector8/2 -> Errors Fo/2  "<evReal>"
  Bus Selector7/4 -> Lo Vel Error/1  "<evReal>"
  Bus Selector6/4 -> Ld Vel Error/1  "<evReal>"

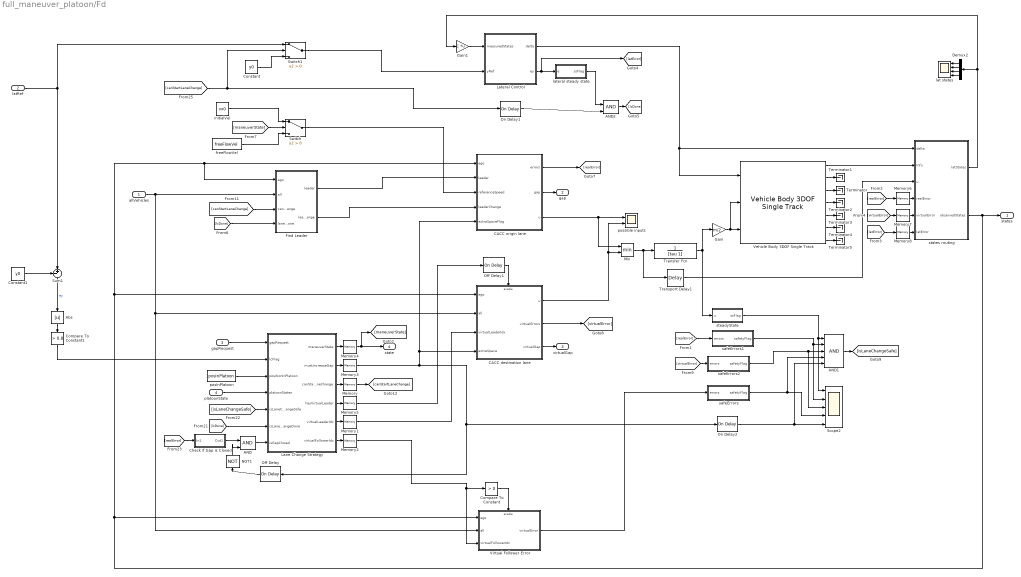
== system full_maneuver_platoon/Fd ==
  allVehicles : Inport
  latRef : Inport  Port=2
  gapRequest : Inport  Port=3
  platoonState : Inport  Port=4
  AND : Logic  IconShape=distinctive  AllPortsSameDT=off  OutDataTypeStr=boolean
  AND1 : Logic  Inputs=5  IconShape=distinctive  AllPortsSameDT=off  OutDataTypeStr=boolean
  AND2 : Logic  IconShape=distinctive  AllPortsSameDT=off  OutDataTypeStr=boolean
  Abs : Abs  SaturateOnIntegerOverflow=off
  CACC destination lane : Subsystem
  CACC origin lane : Subsystem
  Check if Gap is Closed : Subsystem
  Compare To Constant : simulink/Logic and Bit Operations/Compare To Constant  relop=>  const=0  OutDataTypeStr=boolean
  Compare To Constant1 : simulink/Logic and Bit Operations/Compare To Constant  relop=>  const=0.8  OutDataTypeStr=boolean
  Constant : Constant  Value=y0
  Constant1 : Constant  Value=y0
  Demux2 : Demux
  Find Leader : Subsystem
  Gain : Gain  Gain=m/2
  Gain1 : Gain  Gain=C  Multiplication=Matrix(K*u)
  Lane Change Strategy : Subsystem  Variant=on  VariantControlMode=label  LabelModeActiveChoice=leaderFirstInvert
  Lateral Control : Subsystem
  Memory{,1..8} (9 alike) : Memory
  Min : MinMax  Inputs=2
  NOT1 : Logic  Operator=NOT  IconShape=distinctive  AllPortsSameDT=off  OutDataTypeStr=boolean
  Off Delay : powerlib_meascontrol/Logic/On Delay  DelayType=Off delay  delay=1  ic=0  Ts=0
  Off Delay1 : powerlib_meascontrol/Logic/On Delay  DelayType=Off delay  delay=1  ic=0  Ts=0
  On Delay1 : powerlib_meascontrol/Logic/On Delay  DelayType=On delay  delay=1  ic=0  Ts=0
  On Delay2 : powerlib_meascontrol/Logic/On Delay  DelayType=On delay  delay=1  ic=0  Ts=0
  Scope2 : Scope  NumInputPorts=5
  Sum1 : Sum  Inputs=-+|
  Switch : Switch  Criteria=u2 > Threshold  SaturateOnIntegerOverflow=off  InputSameDT=off
  Switch1 : Switch  Criteria=u2 > Threshold  SaturateOnIntegerOverflow=off  InputSameDT=off
  Terminator{,1..5} (6 alike) : Terminator
  Transfer Fcn : TransferFcn  Denominator=[tau 1]
  Transport Delay1 : TransportDelay  DelayTime=0.01
  Vehicle Body 3DOF Single Track : autolibshared/Vehicle Body 3DOF Single Track  trackMode=Single (bicycle)  inputMode=External longitudinal forces  frontSteerMode=on  rearSteerMode=off  windMode=off  muMode=off  extFMode=off  extMMode=off  htchFMode=off  htchMMode=off  extXo=off  extpsio=off  extxdoto=off  extro=off  extYo=off  extTamb=off  extydoto=off  aMode=2  NF=2  NR=2  m=m  a=lf  b=lr  h=0.35  dh=1  hh=0.2  X_o=x0  xdot_o=vx0  CalphaMode=off  sigmaMode=on  d=0  hl=0  w=[1.4,1.4]  Cy_f=12e3  Cy_r=11e3  sigma_f=.1  sigma_r=.1  alpha_f_brk=[-.1 .1]  Cy_f_data=[-9e3 9e3]  alpha_r_brk=[-.1 .1]  Cy_r_data=[-9e3 9e3]  Y_o=y0  ydot_o=0  Izz=4000  psi_o=0  r_o=0  Af=2  Cd=.3  Cl=.1  Cpm=.1  beta_w=[0:0.01:0.3]  Cs=[0:0.03:0.9]  Cym=[0:0.01:0.3]  Pabs=101325  Tair=273  g=9.81  mu=1  xdot_tol=.01  Fznom=5000  Fxtire_sat=7e4  Fytire_sat=7e4  longOff=0  latOff=0  vertOff=0  wrapAng=off
      settings: SourceProductBaseCode=PW,DR,MT,VE
  Virtual Follower Error : Subsystem  TreatAsAtomicUnit=on
  freeFlowVel : Constant  Value=freeFlowVel
  initialVel : Constant  Value=vx0
  lat states : Scope  NumInputPorts=4
  lateral steady state : Subsystem
  posInPlatoon : Constant  Value=posInPlatoon
  possible inputs : Scope  NumInputPorts=2
  safeErrors : Subsystem
  safeErrors1 : Subsystem
  safeErrors2 : Subsystem
  states routing : Subsystem
  steadyState : Subsystem
  states : Outport  VectorParamsAs1DForOutWhenUnconnected=off
  gap : Outport  Port=2  VectorParamsAs1DForOutWhenUnconnected=off
  virtualGap : Outport  Port=3  VectorParamsAs1DForOutWhenUnconnected=off
  state : Outport  Port=4  VectorParamsAs1DForOutWhenUnconnected=off
  wires:
  [virtualError] -> Memory7/1
  [realError] -> Memory6/1
  [latError] -> Memory8/1
  Lane Change Strategy/4(hasVirtualLeader) -> Memory5/1
  Constant1/1 -> Sum1/1
  Memory3/1 -> CACC origin lane/5(extraSpaceFlag), CACC destination lane/4(extraSpace), Off Delay/1, On Delay2/1
  Find Leader/2(leaderChange) -> CACC origin lane/4(leaderChange)
  Find Leader/1(leader) -> CACC origin lane/2(leader)
  Memory5/1 -> Off Delay1/1
  Compare To Constant/1 -> Virtual Follower Error/Enable
  On Delay1/1 -> AND2/2
  lateral steady state/1(ssFlag) -> AND2/1
  Switch1/1 -> Lateral Control/2(yRef)
  [canStartLaneChange] -> On Delay1/1, Switch1/2
  Lateral Control/2(ey) -> lateral steady state/1(e), [latError]
  AND2/1 -> [lcDone]
  Constant/1 -> Switch1/3
  latRef/1 -> Switch1/1, Sum1/2
  Off Delay1/1 -> CACC destination lane/Enable
  Off Delay/1 -> NOT1/1
  NOT1/1 -> AND/2
  Switch/1 -> CACC origin lane/3(referenceSpeed)
  initialVel/1 -> Switch/1
  freeFlowVel/1 -> Switch/3
  [maneuverState] -> Switch/2
  On Delay2/1 -> AND1/5, Scope2/5
  Memory4/1 -> [maneuverState], state/1
  Memory/1 -> [canStartLaneChange]
  safeErrors/1(safetyFlag) -> AND1/4, Scope2/4
  AND1/1 -> [isLaneChangeSafe]
  safeErrors2/1(safetyFlag) -> AND1/3, Scope2/3
  steadyState/1(ssFlag) -> AND1/1, Scope2/1
  safeErrors1/1(safetyFlag) -> AND1/2, Scope2/2
  [virtualError] -> safeErrors2/1(errors)
  [realError] -> safeErrors1/1(errors)
  Virtual Follower Error/1(virtualError) -> safeErrors/1(errors)
  CACC destination lane/3(virtualGap) -> virtualGap/1
  CACC destination lane/2(virtualErrors) -> [virtualError]
  Memory1/1 -> CACC destination lane/3(virtualLeaderIdx)
  CACC destination lane/1(u) -> Min/2, possible inputs/2
  CACC origin lane/2(gap) -> gap/1
  CACC origin lane/1(errors) -> [realError]
  [lcDone] -> Find Leader/4(laneChangeDone)
  [canStartLaneChange] -> Find Leader/3(canStartLaneChange)
  CACC origin lane/3(u) -> possible inputs/1, Min/1
  AND/1 -> Lane Change Strategy/7(isGapClosed)
  Lane Change Strategy/6(virtualFollowerIdx) -> Memory2/1
  Lane Change Strategy/5(virtualLeaderIdx) -> Memory1/1
  Lane Change Strategy/3(canStartLaneChange) -> Memory/1
  Lane Change Strategy/2(mustIncreaseGap) -> Memory3/1
  Lane Change Strategy/1(maneuverState) -> Memory4/1
  Check if Gap is Closed/1(Out1) -> AND/1
  [realError] -> Check if Gap is Closed/1(In1)
  [isLaneChangeSafe] -> Lane Change Strategy/5(isLaneChangeSafe)
  [lcDone] -> Lane Change Strategy/6(isLaneChangeDone)
  posInPlatoon/1 -> Lane Change Strategy/3(positionInPlatoon)
  Compare To Constant1/1 -> Lane Change Strategy/2(lcFlag)
  Transport Delay1/1 -> states routing/3(u)
  Min/1 -> Transfer Fcn/1, Transport Delay1/1
  Vehicle Body 3DOF Single Track/7 -> Terminator5/1
  Vehicle Body 3DOF Single Track/6 -> Terminator4/1
  Vehicle Body 3DOF Single Track/5 -> Terminator3/1
  Vehicle Body 3DOF Single Track/4 -> Terminator2/1
  Vehicle Body 3DOF Single Track/2 -> Terminator1/1
  Demux2/4 -> lat states/4
  Demux2/3 -> lat states/3
  Demux2/2 -> lat states/2
  Demux2/1 -> lat states/1
  Lateral Control/1(delta) -> states routing/1(delta), Vehicle Body 3DOF Single Track/1
  Gain1/1 -> Lateral Control/1(measuredStates)
  states routing/1(latStates) -> Demux2/1, Gain1/1
  platoonState/1 -> Lane Change Strategy/4(platoonStates)
  allVehicles/1 -> Virtual Follower Error/2(all), CACC destination lane/2(all), Find Leader/2(all)
  Abs/1 -> Compare To Constant1/1
  Gain/1 -> Vehicle Body 3DOF Single Track/2, Vehicle Body 3DOF Single Track/3
  Vehicle Body 3DOF Single Track/1 -> states routing/2(Info)
  Vehicle Body 3DOF Single Track/3 -> Terminator/1
  states routing/2(observedStates) -> CACC destination lane/1(ego), CACC origin lane/1(ego), Find Leader/1(ego), Virtual Follower Error/1(ego), states/1
  Transfer Fcn/1 -> Gain/1, steadyState/1(u)
  Sum1/1 -> Abs/1  "ey"
  gapRequest/1 -> Lane Change Strategy/1(gapRequest)
  Memory2/1 -> Compare To Constant/1, Virtual Follower Error/3(virtualFollowerIdx)
  Memory6/1 -> states routing/4(realError)
  Memory7/1 -> states routing/5(virtualError)
  Memory8/1 -> states routing/6(IatError)

== system full_maneuver_platoon/Fo ==
  allVehicles : Inport
  CACC origin lane : Subsystem
  Constant{,1,3,5..6} (5 alike) : Constant  Value=0
  Constant2 : Constant  Value=freeFlowVel
  Constant4 : Constant  Value=[0; 0]
  Gain : Gain  Gain=m/2
  Memory : Memory
  Terminator{,1..2,9..12} (7 alike) : Terminator
  Transfer Fcn : TransferFcn  Denominator=[tau 1]
  Transport Delay1 : TransportDelay  DelayTime=0.01
  Vehicle Body 3DOF Single Track : autolibshared/Vehicle Body 3DOF Single Track  trackMode=Single (bicycle)  inputMode=External longitudinal forces  frontSteerMode=on  rearSteerMode=off  windMode=off  muMode=off  extFMode=off  extMMode=off  htchFMode=off  htchMMode=off  extXo=off  extpsio=off  extxdoto=off  extro=off  extYo=off  extTamb=off  extydoto=off  aMode=2  NF=2  NR=2  m=m  a=lf  b=lr  h=0.35  dh=1  hh=0.2  X_o=x0  xdot_o=vx0  CalphaMode=off  sigmaMode=on  d=0  hl=0  w=[1.4,1.4]  Cy_f=12e3  Cy_r=11e3  sigma_f=.1  sigma_r=.1  alpha_f_brk=[-.1 .1]  Cy_f_data=[-9e3 9e3]  alpha_r_brk=[-.1 .1]  Cy_r_data=[-9e3 9e3]  Y_o=y0  ydot_o=0  Izz=4000  psi_o=0  r_o=0  Af=2  Cd=.3  Cl=.1  Cpm=.1  beta_w=[0:0.01:0.3]  Cs=[0:0.03:0.9]  Cym=[0:0.01:0.3]  Pabs=101325  Tair=273  g=9.81  mu=1  xdot_tol=.01  Fznom=5000  Fxtire_sat=7e4  Fytire_sat=7e4  longOff=0  latOff=0  vertOff=0  wrapAng=off
      settings: SourceProductBaseCode=PW,DR,MT,VE
  findLeader : Subsystem
  states routing1 : Subsystem
  states : Outport  VectorParamsAs1DForOutWhenUnconnected=off
  gap : Outport  Port=2  VectorParamsAs1DForOutWhenUnconnected=off
  wires:
  Memory/1 -> states routing1/4(realError)
  Constant4/1 -> states routing1/5(virtualError)
  [realError] -> Memory/1
  Constant5/1 -> states routing1/6(IatError)
  Vehicle Body 3DOF Single Track/4 -> Terminator9/1
  Vehicle Body 3DOF Single Track/7 -> Terminator12/1
  Vehicle Body 3DOF Single Track/6 -> Terminator11/1
  Vehicle Body 3DOF Single Track/3 -> Terminator/1
  Vehicle Body 3DOF Single Track/5 -> Terminator10/1
  Vehicle Body 3DOF Single Track/2 -> Terminator2/1
  states routing1/1(latStates) -> Terminator1/1
  Constant6/1 -> findLeader/3(lcFlag)
  Constant1/1 -> findLeader/4(state)
  CACC origin lane/2(gap) -> gap/1
  allVehicles/1 -> findLeader/2(all)
  Gain/1 -> Vehicle Body 3DOF Single Track/3, Vehicle Body 3DOF Single Track/2
  Vehicle Body 3DOF Single Track/1 -> states routing1/2(Info)
  states routing1/2(observedStates) -> findLeader/1(ego), CACC origin lane/1(ego), states/1
  Transport Delay1/1 -> states routing1/3(u), Transfer Fcn/1
  findLeader/2(leaderChange) -> CACC origin lane/4(leaderChange)
  CACC origin lane/3(u) -> Transport Delay1/1  "u"
  CACC origin lane/1(errors) -> [realError]
  Constant/1 -> Vehicle Body 3DOF Single Track/1, states routing1/1(delta)  "delta"
  Constant3/1 -> CACC origin lane/5(extraSpaceFlag)
  findLeader/1(leader) -> CACC origin lane/2(leader)
  Transfer Fcn/1 -> Gain/1
  Constant2/1 -> CACC origin lane/3(referenceSpeed)

== system full_maneuver_platoon/Ld ==
  allVehicles : Inport
  CACC origin lane : Subsystem
  Constant{,1,3,5..6} (5 alike) : Constant  Value=0
  Constant2 : Constant  Value=freeFlowVel
  Constant4 : Constant  Value=[0; 0]
  Gain : Gain  Gain=m/2
  Memory : Memory
  Terminator{,1..2,9..12} (7 alike) : Terminator
  Transfer Fcn : TransferFcn  Denominator=[tau 1]
  Transport Delay1 : TransportDelay  DelayTime=0.01
  Vehicle Body 3DOF Single Track : autolibshared/Vehicle Body 3DOF Single Track  trackMode=Single (bicycle)  inputMode=External longitudinal forces  frontSteerMode=on  rearSteerMode=off  windMode=off  muMode=off  extFMode=off  extMMode=off  htchFMode=off  htchMMode=off  extXo=off  extpsio=off  extxdoto=off  extro=off  extYo=off  extTamb=off  extydoto=off  aMode=2  NF=2  NR=2  m=m  a=lf  b=lr  h=0.35  dh=1  hh=0.2  X_o=x0  xdot_o=vx0  CalphaMode=off  sigmaMode=on  d=0  hl=0  w=[1.4,1.4]  Cy_f=12e3  Cy_r=11e3  sigma_f=.1  sigma_r=.1  alpha_f_brk=[-.1 .1]  Cy_f_data=[-9e3 9e3]  alpha_r_brk=[-.1 .1]  Cy_r_data=[-9e3 9e3]  Y_o=y0  ydot_o=0  Izz=4000  psi_o=0  r_o=0  Af=2  Cd=.3  Cl=.1  Cpm=.1  beta_w=[0:0.01:0.3]  Cs=[0:0.03:0.9]  Cym=[0:0.01:0.3]  Pabs=101325  Tair=273  g=9.81  mu=1  xdot_tol=.01  Fznom=5000  Fxtire_sat=7e4  Fytire_sat=7e4  longOff=0  latOff=0  vertOff=0  wrapAng=off
      settings: SourceProductBaseCode=PW,DR,MT,VE
  findLeader : Subsystem
  states routing1 : Subsystem
  states : Outport  VectorParamsAs1DForOutWhenUnconnected=off
  gap : Outport  Port=2  VectorParamsAs1DForOutWhenUnconnected=off
  wires:
  Memory/1 -> states routing1/4(realError)
  Constant4/1 -> states routing1/5(virtualError)
  [realError] -> Memory/1
  Constant5/1 -> states routing1/6(IatError)
  Vehicle Body 3DOF Single Track/4 -> Terminator9/1
  Vehicle Body 3DOF Single Track/7 -> Terminator12/1
  Vehicle Body 3DOF Single Track/6 -> Terminator11/1
  Vehicle Body 3DOF Single Track/3 -> Terminator/1
  Vehicle Body 3DOF Single Track/5 -> Terminator10/1
  Vehicle Body 3DOF Single Track/2 -> Terminator2/1
  states routing1/1(latStates) -> Terminator1/1
  Constant6/1 -> findLeader/3(lcFlag)
  Constant1/1 -> findLeader/4(state)
  CACC origin lane/2(gap) -> gap/1
  allVehicles/1 -> findLeader/2(all)
  Gain/1 -> Vehicle Body 3DOF Single Track/3, Vehicle Body 3DOF Single Track/2
  Vehicle Body 3DOF Single Track/1 -> states routing1/2(Info)
  states routing1/2(observedStates) -> findLeader/1(ego), CACC origin lane/1(ego), states/1
  Transport Delay1/1 -> states routing1/3(u), Transfer Fcn/1
  findLeader/2(leaderChange) -> CACC origin lane/4(leaderChange)
  CACC origin lane/3(u) -> Transport Delay1/1  "u"
  CACC origin lane/1(errors) -> [realError]
  Constant/1 -> Vehicle Body 3DOF Single Track/1, states routing1/1(delta)  "delta"
  Constant3/1 -> CACC origin lane/5(extraSpaceFlag)
  findLeader/1(leader) -> CACC origin lane/2(leader)
  Transfer Fcn/1 -> Gain/1
  Constant2/1 -> CACC origin lane/3(referenceSpeed)

== system full_maneuver_platoon/Lo ==
  allVehicles : Inport
  CACC origin lane : Subsystem
  Constant{,1,3,5..6} (5 alike) : Constant  Value=0
  Constant2 : Constant  Value=freeFlowVel
  Constant4 : Constant  Value=[0; 0]
  Gain : Gain  Gain=m/2
  Memory : Memory
  Terminator{,1..2,9..12} (7 alike) : Terminator
  Transfer Fcn : TransferFcn  Denominator=[tau 1]
  Transport Delay1 : TransportDelay  DelayTime=0.01
  Vehicle Body 3DOF Single Track : autolibshared/Vehicle Body 3DOF Single Track  trackMode=Single (bicycle)  inputMode=External longitudinal forces  frontSteerMode=on  rearSteerMode=off  windMode=off  muMode=off  extFMode=off  extMMode=off  htchFMode=off  htchMMode=off  extXo=off  extpsio=off  extxdoto=off  extro=off  extYo=off  extTamb=off  extydoto=off  aMode=2  NF=2  NR=2  m=m  a=lf  b=lr  h=0.35  dh=1  hh=0.2  X_o=x0  xdot_o=vx0  CalphaMode=off  sigmaMode=on  d=0  hl=0  w=[1.4,1.4]  Cy_f=12e3  Cy_r=11e3  sigma_f=.1  sigma_r=.1  alpha_f_brk=[-.1 .1]  Cy_f_data=[-9e3 9e3]  alpha_r_brk=[-.1 .1]  Cy_r_data=[-9e3 9e3]  Y_o=y0  ydot_o=0  Izz=4000  psi_o=0  r_o=0  Af=2  Cd=.3  Cl=.1  Cpm=.1  beta_w=[0:0.01:0.3]  Cs=[0:0.03:0.9]  Cym=[0:0.01:0.3]  Pabs=101325  Tair=273  g=9.81  mu=1  xdot_tol=.01  Fznom=5000  Fxtire_sat=7e4  Fytire_sat=7e4  longOff=0  latOff=0  vertOff=0  wrapAng=off
      settings: SourceProductBaseCode=PW,DR,MT,VE
  findLeader : Subsystem
  states routing1 : Subsystem
  states : Outport  VectorParamsAs1DForOutWhenUnconnected=off
  gap : Outport  Port=2  VectorParamsAs1DForOutWhenUnconnected=off
  wires:
  Constant2/1 -> CACC origin lane/3(referenceSpeed)
  Transfer Fcn/1 -> Gain/1
  findLeader/1(leader) -> CACC origin lane/2(leader)
  Constant3/1 -> CACC origin lane/5(extraSpaceFlag)
  Constant/1 -> states routing1/1(delta), Vehicle Body 3DOF Single Track/1  "delta"
  CACC origin lane/1(errors) -> [realError]
  CACC origin lane/3(u) -> Transport Delay1/1  "u"
  findLeader/2(leaderChange) -> CACC origin lane/4(leaderChange)
  Transport Delay1/1 -> Transfer Fcn/1, states routing1/3(u)
  states routing1/2(observedStates) -> states/1, CACC origin lane/1(ego), findLeader/1(ego)
  Vehicle Body 3DOF Single Track/1 -> states routing1/2(Info)
  Gain/1 -> Vehicle Body 3DOF Single Track/2, Vehicle Body 3DOF Single Track/3
  allVehicles/1 -> findLeader/2(all)
  CACC origin lane/2(gap) -> gap/1
  Constant1/1 -> findLeader/4(state)
  Constant6/1 -> findLeader/3(lcFlag)
  states routing1/1(latStates) -> Terminator1/1
  Vehicle Body 3DOF Single Track/2 -> Terminator2/1
  Vehicle Body 3DOF Single Track/5 -> Terminator10/1
  Vehicle Body 3DOF Single Track/3 -> Terminator/1
  Vehicle Body 3DOF Single Track/6 -> Terminator11/1
  Vehicle Body 3DOF Single Track/7 -> Terminator12/1
  Vehicle Body 3DOF Single Track/4 -> Terminator9/1
  Constant5/1 -> states routing1/6(IatError)
  [realError] -> Memory/1
  Constant4/1 -> states routing1/5(virtualError)
  Memory/1 -> states routing1/4(realError)
